simulink model "sgAntiSwing"  (R2021b)
settings: Solver=ode4  StartTime=0.0  StopTime=inf  FixedStep=Ts  RelTol=1e-3  EnableMultiTasking=on
model workspace (MAT data in the model file):
  Ts = 0.001
undefined symbols (not defined in the file or in its folder): KD2, N2, Ref, Zero
libraries: slrealtimeutilitieslib x3, slrealtimeiplib x3, slpidlib x2
settings Model: Creator=ronnyl10  LastModifiedBy=jojoa
settings SolverCC: ConcurrentTasks=on  AlgebraicLoopSolver=TrustRegion  PositivePriorityOrder=on  InsertRTBMode=Never (minimum delay)
settings DataIOCC: ExternalInput=ds  SaveFormat=Array  SaveState=on  SignalLoggingName=logsOut
settings OptimizationCC: BlockReduction=off  BooleanDataType=off  OptimizeBlockIOStorage=off  BufferReuse=off  GlobalBufferReuse=off  ExpressionFolding=off  LocalBlockOutputs=off  InitFltsAndDblsToZero=on  OptimizeDataStoreBuffers=off  BusAssignmentInplaceUpdate=off
settings DebuggingCC: SaveWithParameterizedLinksMsg=none  UnderspecifiedInitializationDetection=Classic  MergeDetectMultiDrivingBlocksExec=none  CheckExecutionContextPreStartOutputMsg=on  SignalResolutionControl=TryResolveAllWithWarning  TasksWithSamePriorityMsg=none  SFUnexpectedBacktrackingDiag=warning  SFNoUnconditionalDefaultTransitionDiag=warning  SFExecutionAtInitializationDiag=none  SFMachineParentedDataDiag=warning  ArithmeticOperatorsInVariantConditions=warning
settings HardwareCC: ProdBitPerLong=64  ProdLongLongMode=on  ProdHWDeviceType=Intel->x86-64 (Linux 64)
settings ModelReferenceCC: PropagateSignalLabelsOutOfModel=off
settings SFSimCC: SimUseLocalCustomCode=off  SimTargetLang=C++
settings RTWCC: Description=Simulink Real-Time  SystemTargetFile=slrealtime.tlc  TemplateMakefile=slrealtime_default_tmf  RTWVerbose=off  RTWUseLocalCustomCode=off  Toolchain=Simulink Real-Time Toolchain  BuildConfiguration=Faster Runs  CodeExecutionProfiling=on  TargetLang=C++
settings CodeAppCC: StateflowObjectComments=on
settings SimulinkRealTimeTargetCC: MATLABClassNameForMDSCustomization=Simulink.SoftwareTarget.GRTCustomization  UseGCCFastMath=on
settings ConfigComp: CovMetricSettings=dw  CovSaveCumulativeToWorkspaceVar=on  CovSaveSingleToWorkspaceVar=on  CovExternalEMLEnable=off  CovSFcnEnable=off

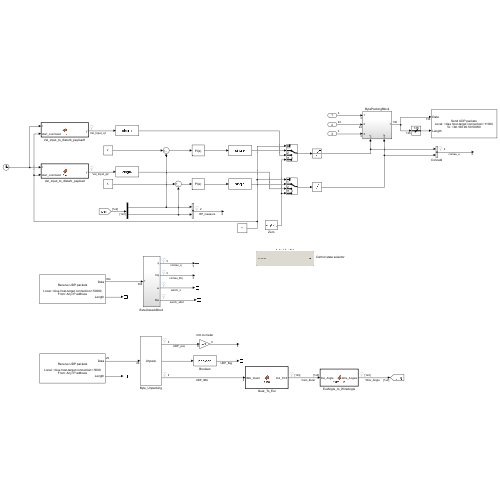
[thumbnail: Simulink's stored preview of the top-level diagram]
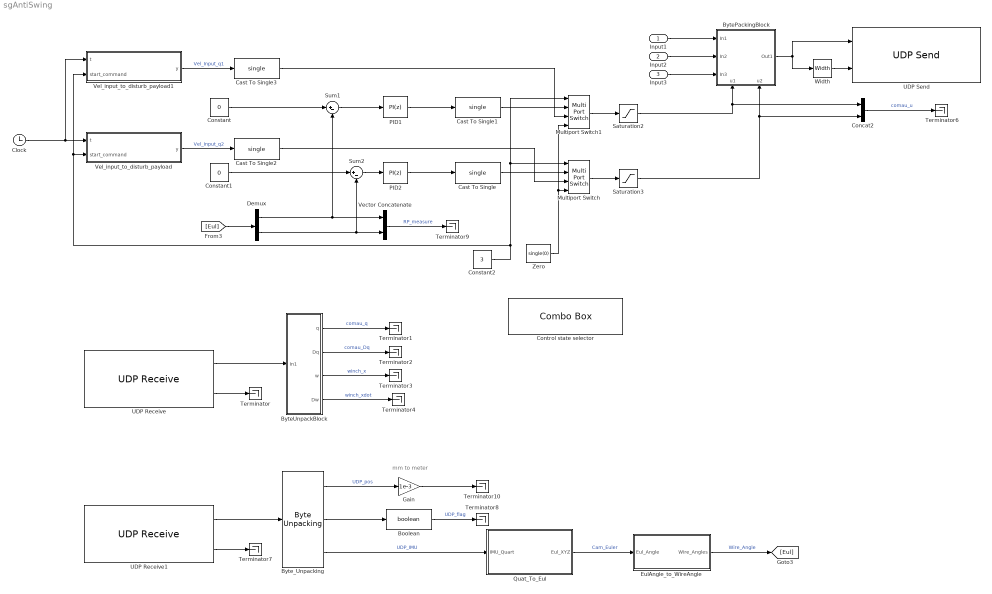
== system sgAntiSwing ==
  note: mm to meter
  Input1 : Inport  OutDataTypeStr=uint32
  Input2 : Inport  Port=2  OutDataTypeStr=single
  Input3 : Inport  Port=3  OutDataTypeStr=single
  Boolean : DataTypeConversion  OutDataTypeStr=boolean
  BytePackingBlock : Subsystem
      settings: PortSchema="{\"entries\":[{\"content\":{\"sides\":[{\"content\":{\"connectorIds\":[\"In1\",\"In2\",\"In3\"]},\"type\":\"ConnectorPlacement.EquallySpacedRectSide\",\"uuid\":\"2ce4a3a0-ffcc-43d7-9a0a-8eda699e79f7\"},{\"content\":{\"connectorIds\":[\"Out1\"],\"side\":\"RIGHT\"},\"type\":\"ConnectorPlacement.EquallySpacedRectSide\",\"uuid\":\"6b0835cb-1c02-4104-b44f-3bd25ad1f1a4\"},{\"content\":{\"connectorIds\":[],\"side\":\"TOP\"},\"type\":\"ConnectorPlacement.EquallySpacedRectSide\",\"uuid\":\"5708f016-a603-4602-bfb0-c60eac1ca3fe\"},{\"content\":{\"connectorIds\":[\"In4\",\"In5\"],\"side\":\"BOTTOM\"},\"type\":\"ConnectorPlacement.EquallySpacedRectSide\",\"uuid\":\"ec76ed57-869b-40d0-9db7-9ec796597bae\"}]},\"type\":\"ConnectorPlacement.EquallySpacedConnector\",\"uuid\":\"dfe3046e-e9d4-4a64-bd13-28ebfaf09d3c\"}],\"packageUris\":[\"http://schema.mathworks.com/mf0/Connector/R2020b\"],\"version\":\"1.0\"}"
  ByteUnpackBlock : Subsystem
  Byte_Unpacking : slrealtimeutilitieslib/Byte Unpacking  MaskUnpackedDataTypes={'int16', 'uint8', 'single'}  MaskUnpackedDataSizes={[6], [1], [4]}  MaskAlignment=1
      settings: SourceProductBaseCode=XP
  Cast To Single{,1..3} (4 alike) : DataTypeConversion  OutDataTypeStr=single
  Clock : Clock
  Concat2 : Concatenate  ConcatenateDimension=2
  Constant : Constant  Value=0
  Constant1 : Constant  Value=0
  Constant2 : Constant  Value=3
  Control state selector : ComboBox  SelectedLabel=Zero-Ref
      settings: Values={{'Zero-Ref', 'Anti-Swing', 'Init Vel Input'}, [3 1 2]}
  Demux : Demux  Outputs=2
  EulAngle_to_WireAngle : MATLAB Function  TreatAsAtomicUnit=on
  Gain : Gain  Gain=1e-3
  Multiport Switch : MultiPortSwitch
  Multiport Switch1 : MultiPortSwitch
  PID1 : slpidlib/PID Controller  Controller=PI  Form=Parallel  TimeDomain=Discrete-time  UseExternalTs=off  SampleTime=-1  IntegratorMethod=Forward Euler  FilterMethod=Forward Euler  ControllerParametersSource=internal  P=0.015  I=0  D=KD2  UseFilter=on  N=N2  TunerSelectOption=Transfer Function Based (PID Tuner App)  InitialConditionSource=internal  InitialConditionForIntegrator=0  InitialConditionForFilter=0  DifferentiatorICPrevScaledInput=0  ExternalReset=none  TrackingMode=off  Kt=1  LimitOutput=off  SatLimitsSource=internal  UpperSaturationLimit=inf  LowerSaturationLimit=-inf  LinearizeAsGain=on  AntiWindupMode=none  Kb=1  POutMin=[]  POutMax=[]  IOutMin=[]  IOutMax=[]  DOutMin=[]  DOutMax=[]  NOutMin=[]  NOutMax=[]  SumOutMin=[]  SumOutMax=[]  SaturationOutMin=[]  SaturationOutMax=[]  PParamMin=[]  PParamMax=[]  IParamMin=[]  IParamMax=[]  DParamMin=[]  DParamMax=[]  NParamMin=[]  NParamMax=[]  KbParamMin=[]  KbParamMax=[]  KtParamMin=[]  KtParamMax=[]  KbOutMin=[]  KbOutMax=[]  KtOutMin=[]  KtOutMax=[]  IntegratorOutMin=[]  IntegratorOutMax=[]  FilterOutMin=[]  FilterOutMax=[]  SumI1OutMin=[]  SumI1OutMax=[]  SumI2OutMin=[]  SumI2OutMax=[]  SumI3OutMin=[]  SumI3OutMax=[]  SumI4OutMin=[]  SumI4OutMax=[]  SumDOutMin=[]  SumDOutMax=[]  DifferentiatorOutMin=[]  DifferentiatorOutMax=[]  FilterDiffOutCoefMin=[]  FilterDiffOutCoefMax=[]  ReciprocalOutMin=[]  ReciprocalOutMax=[]  SumDenOutMin=[]  SumDenOutMax=[]  SumNumOutMin=[]  SumNumOutMax=[]  DivideOutMin=[]  DivideOutMax=[]  UdiffTsProdOutMin=[]  UdiffTsProdOutMax=[]  NTsProdOutMin=[]  NTsProdOutMax=[]  UintegralTsProdOutMin=[]  UintegralTsProdOutMax=[]  UngainTsProdOutMin=[]  UngainTsProdOutMax=[]  FilterDenConstantOutDataTypeStr=Inherit: Inherit via back propagation  FilterDenConstantOutMin=[]  FilterDenConstantOutMax=[]  PCopyOutDataTypeStr=Inherit: Inherit via back propagation  PCopyOutMin=[]  PCopyOutMax=[]  NCopyOutDataTypeStr=Inherit: Inherit via back propagation  NCopyOutMin=[]  NCopyOutMax=[]  IntegratorContinuousStateAttributes=''  IntegratorStateMustResolveToSignalObject=off  IntegratorRTWStateStorageClass=Auto  FilterContinuousStateAttributes=''  FilterStateMustResolveToSignalObject=off  FilterRTWStateStorageClass=Auto  ParallelPVariant=InternalParameters  IdealPVariant=Disabled  IVariant=InternalParameters  DVariant=Disabled  IntegratorVariant=Discrete  SatVariant=Disabled  AWVariant=Passthrough  PCopyVariant=Disabled  TRVariant=Disabled  FdbkBlocksVariant=Forward  IdealPFdbkVariant=Disabled  SatFdbkVariant=Disabled  DerivativeFilterVariant=Disabled  NVariant=Disabled  NCopyVariant=Disabled_SignalSpec  FilterICVariant=Disabled  IntegratorICVariant=InternalICs  ExternalResetVariant=Disabled  TRSumVariant=Passthrough  SumFdbkVariant=Disabled  SumVariant=Sum_PI  TsampFilterVariant=InternalTs  TsampNgainVariant=Passthrough  TsampIntegralVariant=Passthrough  ExternalSaturationOutDataTypeStr=Inherit: Same as second input
  PID2 : slpidlib/PID Controller  Controller=PI  Form=Parallel  TimeDomain=Discrete-time  UseExternalTs=off  SampleTime=-1  IntegratorMethod=Forward Euler  FilterMethod=Forward Euler  ControllerParametersSource=internal  P=0.015  I=0  D=KD2  UseFilter=on  N=N2  TunerSelectOption=Transfer Function Based (PID Tuner App)  InitialConditionSource=internal  InitialConditionForIntegrator=0  InitialConditionForFilter=0  DifferentiatorICPrevScaledInput=0  ExternalReset=none  TrackingMode=off  Kt=1  LimitOutput=off  SatLimitsSource=internal  UpperSaturationLimit=inf  LowerSaturationLimit=-inf  LinearizeAsGain=on  AntiWindupMode=none  Kb=1  POutMin=[]  POutMax=[]  IOutMin=[]  IOutMax=[]  DOutMin=[]  DOutMax=[]  NOutMin=[]  NOutMax=[]  SumOutMin=[]  SumOutMax=[]  SaturationOutMin=[]  SaturationOutMax=[]  PParamMin=[]  PParamMax=[]  IParamMin=[]  IParamMax=[]  DParamMin=[]  DParamMax=[]  NParamMin=[]  NParamMax=[]  KbParamMin=[]  KbParamMax=[]  KtParamMin=[]  KtParamMax=[]  KbOutMin=[]  KbOutMax=[]  KtOutMin=[]  KtOutMax=[]  IntegratorOutMin=[]  IntegratorOutMax=[]  FilterOutMin=[]  FilterOutMax=[]  SumI1OutMin=[]  SumI1OutMax=[]  SumI2OutMin=[]  SumI2OutMax=[]  SumI3OutMin=[]  SumI3OutMax=[]  SumI4OutMin=[]  SumI4OutMax=[]  SumDOutMin=[]  SumDOutMax=[]  DifferentiatorOutMin=[]  DifferentiatorOutMax=[]  FilterDiffOutCoefMin=[]  FilterDiffOutCoefMax=[]  ReciprocalOutMin=[]  ReciprocalOutMax=[]  SumDenOutMin=[]  SumDenOutMax=[]  SumNumOutMin=[]  SumNumOutMax=[]  DivideOutMin=[]  DivideOutMax=[]  UdiffTsProdOutMin=[]  UdiffTsProdOutMax=[]  NTsProdOutMin=[]  NTsProdOutMax=[]  UintegralTsProdOutMin=[]  UintegralTsProdOutMax=[]  UngainTsProdOutMin=[]  UngainTsProdOutMax=[]  FilterDenConstantOutDataTypeStr=Inherit: Inherit via back propagation  FilterDenConstantOutMin=[]  FilterDenConstantOutMax=[]  PCopyOutDataTypeStr=Inherit: Inherit via back propagation  PCopyOutMin=[]  PCopyOutMax=[]  NCopyOutDataTypeStr=Inherit: Inherit via back propagation  NCopyOutMin=[]  NCopyOutMax=[]  IntegratorContinuousStateAttributes=''  IntegratorStateMustResolveToSignalObject=off  IntegratorRTWStateStorageClass=Auto  FilterContinuousStateAttributes=''  FilterStateMustResolveToSignalObject=off  FilterRTWStateStorageClass=Auto  ParallelPVariant=InternalParameters  IdealPVariant=Disabled  IVariant=InternalParameters  DVariant=Disabled  IntegratorVariant=Discrete  SatVariant=Disabled  AWVariant=Passthrough  PCopyVariant=Disabled  TRVariant=Disabled  FdbkBlocksVariant=Forward  IdealPFdbkVariant=Disabled  SatFdbkVariant=Disabled  DerivativeFilterVariant=Disabled  NVariant=Disabled  NCopyVariant=Disabled_SignalSpec  FilterICVariant=Disabled  IntegratorICVariant=InternalICs  ExternalResetVariant=Disabled  TRSumVariant=Passthrough  SumFdbkVariant=Disabled  SumVariant=Sum_PI  TsampFilterVariant=InternalTs  TsampNgainVariant=Passthrough  TsampIntegralVariant=Passthrough  ExternalSaturationOutDataTypeStr=Inherit: Same as second input
  Quat_To_Eul : MATLAB Function  TreatAsAtomicUnit=on
  Saturation2 : Saturate  UpperLimit=0.4  LowerLimit=-0.4
  Saturation3 : Saturate  UpperLimit=0.4  LowerLimit=-0.4
  Sum1 : Sum  Inputs=|+-
  Sum2 : Sum  Inputs=|+-
  Terminator{,1..4,6..10} (10 alike) : Terminator
  UDP Receive : slrealtimeiplib/UDP Receive  useHostTargetConn=on  ipAddress=192.168.90.60  localPort=50060  rcvWidth=304  rcvFmAny=on  fmAddress=192.168.90.50  sampleTime=Ts
      settings: SourceProductBaseCode=XP
  UDP Receive1 : slrealtimeiplib/UDP Receive  useHostTargetConn=on  ipAddress=192.168.80.15  localPort=5008  rcvWidth=29  rcvFmAny=on  fmAddress='192.168.80.10'  sampleTime=Ts
      settings: SourceProductBaseCode=XP
  UDP Send : slrealtimeiplib/UDP Send  useHostTargetConn=on  toAddress=192.168.90.50  toPort=50050  sampleTime=Ts  localPort=11000
      settings: SourceProductBaseCode=XP
  Vector Concatenate : Concatenate
  Vel_input_to_disturb_payload : MATLAB Function  TreatAsAtomicUnit=on
  Vel_input_to_disturb_payload1 : MATLAB Function  TreatAsAtomicUnit=on
  Width : Width
  Zero : Constant  Value=single(0)
  wires:
  Width/1 -> UDP Send/2
  UDP Receive/2 -> Terminator/1
  Concat2/1 -> Terminator6/1  "comau_u"
  BytePackingBlock/1(Out1) -> Width/1, UDP Send/1
  Input1/1 -> BytePackingBlock/1(In1)
  Input3/1 -> BytePackingBlock/3(In3)
  Input2/1 -> BytePackingBlock/2(In2)
  UDP Receive/1 -> ByteUnpackBlock/1(In1)
  ByteUnpackBlock/3(w) -> Terminator3/1  "winch_x"
  ByteUnpackBlock/4(Dw) -> Terminator4/1  "winch_xdot"
  Saturation3/1 -> BytePackingBlock/5(u2), Concat2/2
  Saturation2/1 -> BytePackingBlock/4(u1), Concat2/1
  ByteUnpackBlock/2(Dq) -> Terminator2/1  "comau_Dq"
  ByteUnpackBlock/1(q) -> Terminator1/1  "comau_q"
  Boolean/1 -> Terminator8/1  "UDP_flag"
  Byte_Unpacking/3 -> Quat_To_Eul/1(IMU_Quart)  "UDP_IMU"
  Gain/1 -> Terminator10/1
  Byte_Unpacking/1 -> Gain/1  "UDP_pos"
  Byte_Unpacking/2 -> Boolean/1
  UDP Receive1/1 -> Byte_Unpacking/1
  UDP Receive1/2 -> Terminator7/1
  Quat_To_Eul/1(Eul_XYZ) -> EulAngle_to_WireAngle/1(Eul_Angle)  "Cam_Euler"
  EulAngle_to_WireAngle/1(Wire_Angles) -> [Eul]  "Wire_Angle"
  Cast To Single3/1 -> Multiport Switch1/3
  Multiport Switch/1 -> Saturation3/1
  Constant/1 -> Sum1/1
  PID1/1 -> Cast To Single1/1
  [Eul] -> Demux/1
  Cast To Single/1 -> Multiport Switch/2
  Cast To Single2/1 -> Multiport Switch/3
  Sum2/1 -> PID2/1
  Sum1/1 -> PID1/1
  Constant1/1 -> Sum2/1
  Vector Concatenate/1 -> Terminator9/1  "RP_measure"
  Cast To Single1/1 -> Multiport Switch1/2
  Multiport Switch1/1 -> Saturation2/1
  PID2/1 -> Cast To Single/1
  Demux/2 -> Sum2/2, Vector Concatenate/2
  Vel_input_to_disturb_payload/1(y) -> Cast To Single2/1  "Vel_Input_q2"
  Vel_input_to_disturb_payload1/1(y) -> Cast To Single3/1  "Vel_Input_q1"
  Zero/1 -> Multiport Switch1/4, Multiport Switch/4
  Demux/1 -> Sum1/2, Vector Concatenate/1
  Constant2/1 -> Multiport Switch/1, Multiport Switch1/1, Vel_input_to_disturb_payload/2(start_command), Vel_input_to_disturb_payload1/2(start_command)
  Clock/1 -> Vel_input_to_disturb_payload1/1(t), Vel_input_to_disturb_payload/1(t)

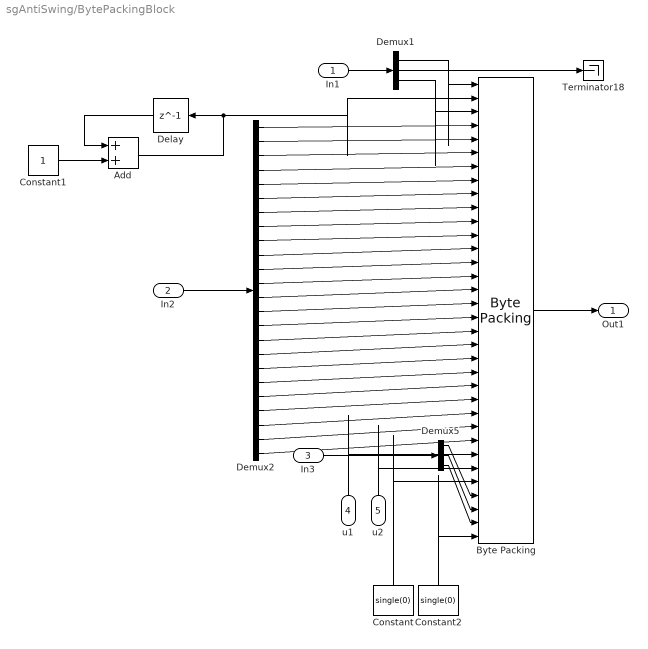
== system sgAntiSwing/BytePackingBlock ==
  In1 : Inport
  In2 : Inport  Port=2
  In3 : Inport  Port=3
  u1 : Inport  Port=4
  u2 : Inport  Port=5
  Add : Sum
  Byte Packing : slrealtimeutilitieslib/Byte Packing  MaskPackedDataType=uint8  MaskUnpackedDataTypes={'uint32', 'uint32', 'uint32', 'single', 'single', 'single', 'single', 'single', 'single', 'single', 'single', 'single', 'single', 'single', 'single', 'single', 'single', 'single', 'single', 'single', 'single', 'single', 'single', 'single', 'single', 'single', 'single', 'single', 'single', 'single', 'single', 'single', 'single', 'single'}  MaskAlignment=1
  Constant : Constant  Value=single(0)
  Constant1 : Constant  OutDataTypeStr=uint32
  Constant2 : Constant  Value=single(0)
  Delay : Delay  DelayLength=1
  Demux1 : Demux  Outputs=3
  Demux2 : Demux  Outputs=24
  Demux5 : Demux  Outputs=3
  Terminator18 : Terminator
  Out1 : Outport
  wires:
  Demux2/19 -> Byte Packing/22
  Demux2/21 -> Byte Packing/24
  Constant/1 -> Byte Packing/30
  Demux2/2 -> Byte Packing/5
  u2/1 -> Byte Packing/29
  Demux5/1 -> Byte Packing/31
  Demux5/2 -> Byte Packing/32
  Demux1/3 -> Byte Packing/3
  In2/1 -> Demux2/1
  Demux2/22 -> Byte Packing/25
  Demux2/1 -> Byte Packing/4
  Demux2/15 -> Byte Packing/18
  Demux2/18 -> Byte Packing/21
  Delay/1 -> Add/1
  Demux2/24 -> Byte Packing/27
  Demux1/2 -> Terminator18/1
  In1/1 -> Demux1/1
  Demux2/5 -> Byte Packing/8
  Add/1 -> Byte Packing/2, Delay/1
  Constant1/1 -> Add/2
  Demux2/6 -> Byte Packing/9
  Demux2/9 -> Byte Packing/12
  Demux2/10 -> Byte Packing/13
  Demux2/20 -> Byte Packing/23
  Demux2/8 -> Byte Packing/11
  Demux2/12 -> Byte Packing/15
  Demux2/23 -> Byte Packing/26
  Demux2/16 -> Byte Packing/19
  Demux1/1 -> Byte Packing/1
  Demux5/3 -> Byte Packing/33
  Demux2/3 -> Byte Packing/6
  Demux2/11 -> Byte Packing/14
  Demux2/7 -> Byte Packing/10
  Demux2/4 -> Byte Packing/7
  Demux2/13 -> Byte Packing/16
  Demux2/17 -> Byte Packing/20
  Demux2/14 -> Byte Packing/17
  u1/1 -> Byte Packing/28
  In3/1 -> Demux5/1
  Byte Packing/1 -> Out1/1
  Constant2/1 -> Byte Packing/34

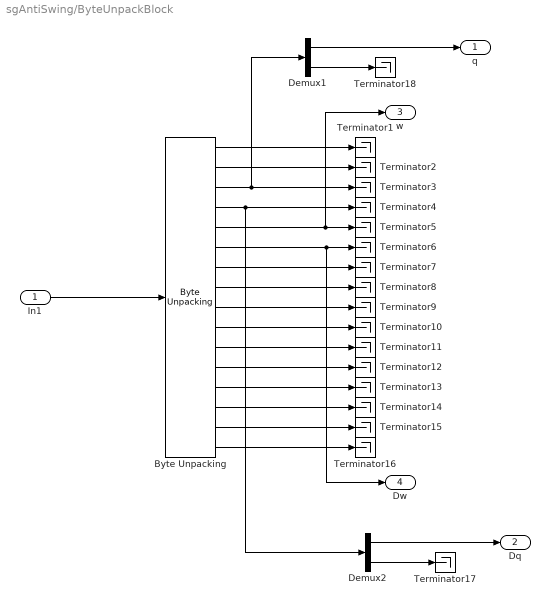
== system sgAntiSwing/ByteUnpackBlock ==
  In1 : Inport
  Byte Unpacking : slrealtimeutilitieslib/Byte Unpacking  MaskUnpackedDataTypes={'uint32', 'single', 'single', 'single', 'single', 'single', 'single', 'single', 'single', 'single', 'single', 'single', 'single', 'single', 'single', 'single'}  MaskUnpackedDataSizes={[1], [1], [6], [6], [1], [1], [6], [6], [6], [6], [6], [6], [6], [6], [6], [6]}  MaskAlignment=1
      settings: SourceProductBaseCode=XP
  Demux1 : Demux  Outputs=2
  Demux2 : Demux  Outputs=2
  Terminator{1..18} (18 alike) : Terminator
  q : Outport
  Dq : Outport  Port=2
  w : Outport  Port=3
  Dw : Outport  Port=4
  wires:
  Byte Unpacking/13 -> Terminator13/1
  Byte Unpacking/8 -> Terminator8/1
  Byte Unpacking/1 -> Terminator1/1
  Byte Unpacking/7 -> Terminator7/1
  Byte Unpacking/16 -> Terminator16/1
  Byte Unpacking/6 -> Terminator6/1, Dw/1
  Byte Unpacking/11 -> Terminator11/1
  Byte Unpacking/10 -> Terminator10/1
  Byte Unpacking/15 -> Terminator15/1
  Byte Unpacking/2 -> Terminator2/1
  Byte Unpacking/14 -> Terminator14/1
  Byte Unpacking/5 -> w/1, Terminator5/1
  Byte Unpacking/9 -> Terminator9/1
  Byte Unpacking/12 -> Terminator12/1
  In1/1 -> Byte Unpacking/1
  Demux1/1 -> q/1
  Byte Unpacking/3 -> Demux1/1, Terminator3/1
  Demux2/1 -> Dq/1
  Byte Unpacking/4 -> Demux2/1, Terminator4/1
  Demux1/2 -> Terminator18/1
  Demux2/2 -> Terminator17/1

== matlab function sgAntiSwing/Quat_To_Eul ==
  data: IMU_Quart input; Eul_XYZ output
function Eul_XYZ  = func(IMU_Quart)
    %Reorder quaternion from luxonis default [x; y; z; w] to matlab default [w, x, y, z]
    temp = IMU_Quart;
    q = [temp(4), temp(1), temp(2), temp(3)];
    
    Eul_XYZ = quat2eul(q);
    Eul_XYZ = rad2deg(Eul_XYZ);
end

== matlab function sgAntiSwing/Vel_input_to_disturb_payload ==
  data: t input; y output; start_command input
function y = fcn(t, start_command)
%#codegen

persistent t_command_received profile_triggered;

if isempty(t_command_received)
    t_command_received = -1;
    profile_triggered = false;
end

% --- Constants ---
peak_value     = 0.2;
total_duration = 2.5;          % total time from start of accel to end of final decel
hold_duration  = 0.25;          % time to hold at +peak and at -peak
ramp_duration  = (total_duration - 2*hold_duration) / 4; 
start_delay    = 0;          % seconds between command and start of profile

% --- Default Output ---
y = 0.0;

% --- Trigger on command == 2 ---
if start_command == 2 && ~profile_triggered
    t_command_received = t;
    profile_triggered   = true;
end

if profile_triggered
    t0 = t_command_received + start_delay;
    if t < t0
        % still in delay
        y = 0;
    else
        t_elapsed = t - t0;
        
        % segment boundaries
        t1 = ramp_duration;
        t2 = t1 + hold_duration;
        t3 = t2 + ramp_duration;
        t4 = t3 + ramp_duration;
        t5 = t4 + hold_duration;
        t6 = t5 + ramp_duration;  % should equal total_duration
        
        if t_elapsed < t1
            % 1) ramp 0 -> +peak
            y = (peak_value / ramp_duration) * t_elapsed;
            
        elseif t_elapsed < t2
            % 2) hold at +peak
            y = peak_value;
            
        elseif t_elapsed < t3
            % 3) ramp +peak -> 0
            y = peak_value + ( -peak_value / ramp_duration ) * (t_elapsed - t2);
            
        elseif t_elapsed < t4
            % 4) ramp 0 -> -peak
            y = 0 + ( -peak_value / ramp_duration ) * (t_elapsed - t3);
            
        elseif t_elapsed < t5
            % 5) hold at -peak
            y = -peak_value;
            
        elseif t_elapsed <= t6
            % 6) ramp -peak -> 0
            y = -peak_value + ( peak_value / ramp_duration ) * (t_elapsed - t5);
            
        else
            % finished
            y = 0;
            % to allow re‑trigger later, you could reset:
            % profile_triggered = false;
        end
    end
end

end

== matlab function sgAntiSwing/Vel_input_to_disturb_payload1 ==
  data: t input; y output; start_command input
function y = fcn(t, start_command)
%#codegen

persistent t_command_received profile_triggered;

if isempty(t_command_received)
    t_command_received = -1;
    profile_triggered = false;
end

% --- Constants ---
peak_value     = 0.2;
total_duration = 2.5;          % total time from start of accel to end of final decel
hold_duration  = 0.25;          % time to hold at +peak and at -peak
ramp_duration  = (total_duration - 2*hold_duration) / 4; 
start_delay    = 2.0;          % seconds between command and start of profile

% --- Default Output ---
y = 0.0;

% --- Trigger on command == 2 ---
if start_command == 2 && ~profile_triggered
    t_command_received = t;
    profile_triggered   = true;
end

if profile_triggered
    t0 = t_command_received + start_delay;
    if t < t0
        % still in delay
        y = 0;
    else
        t_elapsed = t - t0;
        
        % segment boundaries
        t1 = ramp_duration;
        t2 = t1 + hold_duration;
        t3 = t2 + ramp_duration;
        t4 = t3 + ramp_duration;
        t5 = t4 + hold_duration;
        t6 = t5 + ramp_duration;  % should equal total_duration
        
        if t_elapsed < t1
            % 1) ramp 0 -> +peak
            y = (peak_value / ramp_duration) * t_elapsed;
            
        elseif t_elapsed < t2
            % 2) hold at +peak
            y = peak_value;
            
        elseif t_elapsed < t3
            % 3) ramp +peak -> 0
            y = peak_value + ( -peak_value / ramp_duration ) * (t_elapsed - t2);
            
        elseif t_elapsed < t4
            % 4) ramp 0 -> -peak
            y = 0 + ( -peak_value / ramp_duration ) * (t_elapsed - t3);
            
        elseif t_elapsed < t5
            % 5) hold at -peak
            y = -peak_value;
            
        elseif t_elapsed <= t6
            % 6) ramp -peak -> 0
            y = -peak_value + ( peak_value / ramp_duration ) * (t_elapsed - t5);
            
        else
            % finished
            y = 0;
            % to allow re‑trigger later, you could reset:
            % profile_triggered = false;
        end
    end
end

end

== matlab function sgAntiSwing/EulAngle_to_WireAngle ==
  data: Eul_Angle input; Wire_Angles output
function Wire_Angles = Wire_Tilt(Eul_Angle)

    phi_rest_deg = -0.8270;   % Resting Roll angle
    theta_rest_deg = -9.2933; % Resting Pitch angle

    %Deadband zone to ignore IMU disturbances around rest point of wire
    phi_rest_min = -1.25;  %Roll deadzone
    phi_rest_max = -0.85 ;  
    theta_rest_min = -9.5; % Lower bound for Pitch dead zone
    theta_rest_max = -9.0; % Upper bound for Pitch dead zone

    %Measured angles of roll and pitch
    pitch_meas_deg = Eul_Angle(2);
    roll_meas_deg = Eul_Angle(3);

    % Initialize output vector
    Wire_Angles = [0.0, 0.0];

    %Calculate Front View Angle (from Roll) with Dead Zone
    if (roll_meas_deg >= phi_rest_min && roll_meas_deg <= phi_rest_max)
        % Measurement is within the resting range uncertainty - keep angle as zero
        Wire_Angles(1) = 0.0;
    else
        %Measurement is outside the range - calculate deviation from the center rest angle
        Wire_Angles(1) = roll_meas_deg - phi_rest_deg;
    end

    %Calculate Side View Angle (from Pitch) with Dead Zone
    if (pitch_meas_deg >= theta_rest_min && pitch_meas_deg <= theta_rest_max)
        % Measurement is within the resting range uncertainty - keep angle as zero
        Wire_Angles(2) = 0.0;
    else
        %Measurement is outside the range - calculate deviation from the center rest angle
        Wire_Angles(2) = pitch_meas_deg - theta_rest_deg;
    end

    % Output Wire_Angles contains [FrontViewAngle_deg, SideViewAngle_deg]
end
